simulink model "Const_VF_WithSlipCompensation"  (R2023a)
settings: Solver=VariableStepAuto  StartTime=0.0  StopTime=10.0  RelTol=1e-3
values from neighbouring files (symbols this model uses):
  Lm = .2037    (= 0.2037)    [Parameters.m]
  offset = Vph_p-(slope*Freq)    [Parameters.m]
  P = 4    [Parameters.m]
  slope = (Vph_p-VF_boost)/(Freq-1)    [Parameters.m]
  Te_rated = Prated/Wr_rated    (= 20.3536435794)    [Parameters.m]
  Vph_p = VLL_p/sqrt(3)    [Parameters.m]
  Wslip_rated = Ws_rated-Wr_rated    (= 5.23598775598)    [Parameters.m]
libraries: spsMosfetLib x6, spsabctodq0Lib x2, spsAsynchronousMachineSIUnitsLib x1, spsCurrentMeasurementLib x1, spsDCVoltageSourceLib x1, spsTriangleGeneratorLib x1, sps_lib x1
settings Model: Creator=User  LastModifiedBy=User

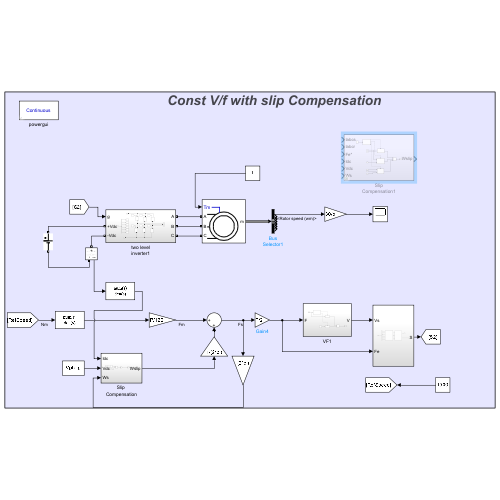
[thumbnail: Simulink's stored preview of the top-level diagram]
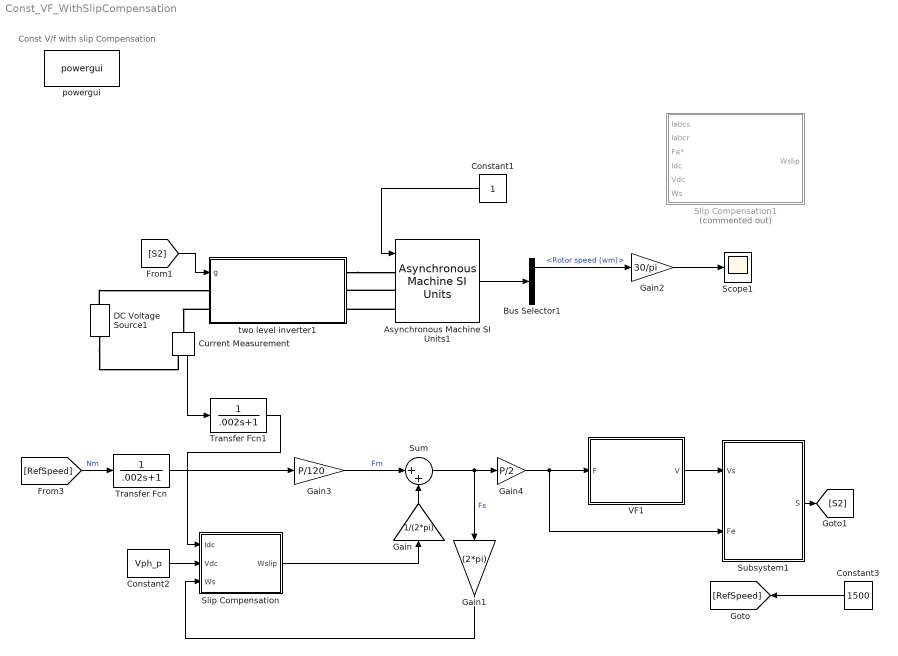
== system Const_VF_WithSlipCompensation ==
  note: Const V/f with slip Compensation
  Asynchronous Machine SI Units1 : spsAsynchronousMachineSIUnitsLib/Asynchronous Machine SI Units  RotorType=Squirrel-cage  PresetModel="01:  5 HP   460 V 60Hz 1750 RPM"  MechanicalLoad=Torque Tm  ShowDetailedParameters=on  ReferenceFrame=Stationary  Units=SI  MeasurementBus=off  NominalParameters=[3730 460 60]  VoltageRatio=1  Stator=[1.115 0.005974]  Rotor=[1.083 0.005974]  Cage1=[0.4155 0.002066]  Cage2=[0.4168 0.0003495]  Lm=0.2037  Mechanical=[0.02 0.005752 2]  PolePairs=2  InitialConditions=[1 0 0 0 0 0 0 0]  SimulateSaturation=off  Saturation=[14.03593122, 27.81365428, 53.79336849, 72.68890987, 97.98006896, 148.6815601, 215.7428561, 302.9841135, 428.7778367 ; 230, 322, 414, 460, 506, 552, 598, 644, 690]  LoadFlowParameters=1492000  TsPowergui=0  TsBlock=-1  IterativeModel=Trapezoidal non iterative  IterativeDiscreteModel=Trapezoidal non iterative  Pmec=1.492e+006
  Bus Selector1 : BusSelector  OutputSignals=Mechanical.Rotor speed (wm),Stator measurements.Stator current is_a (A),Stator measurements.Stator current is_b (A),Stator measurements.Stator current is_c (A),Rotor measurements.Rotor current ir_a (A),Rotor measurements.Rotor current ir_b (A),Rotor measurements.Rotor current ir_c (A)
  Constant1 : Constant
  Constant2 : Constant  Value=Vph_p
  Constant3 : Constant  Value=1500
  Current Measurement : spsCurrentMeasurementLib/Current Measurement  PhasorSimulation=off  OutputType=Complex  PSBequivalent=0
  DC Voltage Source1 : spsDCVoltageSourceLib/DC Voltage Source  Amplitude=Vph_p  Measurements=None
  Gain : Gain  Gain=1/(2*pi)
  Gain1 : Gain  Gain=(2*pi)
  Gain2 : Gain  Gain=30/pi
  Gain3 : Gain  Gain=P/120
  Gain4 : Gain  Gain=P/2
  Scope1 : Scope
  Slip Compensation1 : Subsystem  Commented=on
  Slip Compensation : Subsystem
  Subsystem1 : Subsystem
  Sum : Sum  Inputs=|++
  Transfer Fcn : TransferFcn  Denominator=[.002 1]
  Transfer Fcn1 : TransferFcn  Denominator=[.002 1]
  VF1 : Subsystem
  powergui : sps_lib/powergui  Priority=1  SimulationMode=Continuous  SampleTime=50e-6  frequency=60  Iterations=50  frequencyindice=60  Pbase=100e6  ErrMax=1e-4  UnitsV=kV  UnitsW=MW  buscounter=0  FunctionMessages=off  echomessages=off  EnableUseOfTLC=off  CurrentSourceSwitches=off  DisableSnubberDevices=off  DisableRonSwitches=off  DisableVfSwitches=off  DisplayEquations=off  AutomaticDiscreteSolvers=off  SolverType=Tustin/Backward Euler (TBE)  Interpol=off  ExternalGateDelay=off  methode=off  Ts=100  x0status=blocks  SPID=on  SwTol=0  HookPort=off  NonlinearTolerance=1e-4  nMaxIteration=100  ContinueOnMaxIteration=off  RestoreLinks=warning  ResistiveCurrentMeasurement=off  Frange=[0:2:500]  Ylog=off  Xlog=on  ShowGrid=off  save=off  variable=ZData  structure=0  ZoomFFT=off  StartTime=0.0  cycles=1  DisplayStyle=1  fundamental=60  FreqAxis=off  MaxFrequency=1000  frequencyindicesteady=1  RmsSteady=1  display=off
  two level inverter1 : Subsystem
  wires:
  Subsystem1/1(S) -> [S2]
  Gain3/1 -> Sum/1  "Fm"
  Gain2/1 -> Scope1/1
  Constant1/1 -> Asynchronous Machine SI Units1/1
  Sum/1 -> Gain4/1, Gain1/1  "Fs"
  [RefSpeed] -> Transfer Fcn/1  "Nm"
  [S2] -> two level inverter1/1(g)
  Asynchronous Machine SI Units1/1 -> Bus Selector1/1
  Bus Selector1/1 -> Gain2/1  "<Rotor speed (wm)>"
  VF1/1(V) -> Subsystem1/1(Vs)
  Constant3/1 -> [RefSpeed]
  Gain/1 -> Sum/2
  Gain4/1 -> Subsystem1/2(Fe), VF1/1(F)
  Transfer Fcn/1 -> Gain3/1
  Constant2/1 -> Slip Compensation/2(Vdc)
  Current Measurement/1 -> Transfer Fcn1/1
  Gain1/1 -> Slip Compensation/3(Ws)
  Transfer Fcn1/1 -> Slip Compensation/1(Idc)
  Slip Compensation/1(Wslip) -> Gain/1
  connections:
  DC Voltage Source1/RConn1 -- two level inverter1/LConn1
  two level inverter1/RConn1 -- Asynchronous Machine SI Units1/LConn1
  Asynchronous Machine SI Units1/LConn3 -- two level inverter1/RConn3
  DC Voltage Source1/LConn1 -- Current Measurement/RConn1
  Asynchronous Machine SI Units1/LConn2 -- two level inverter1/RConn2
  two level inverter1/LConn2 -- Current Measurement/LConn1

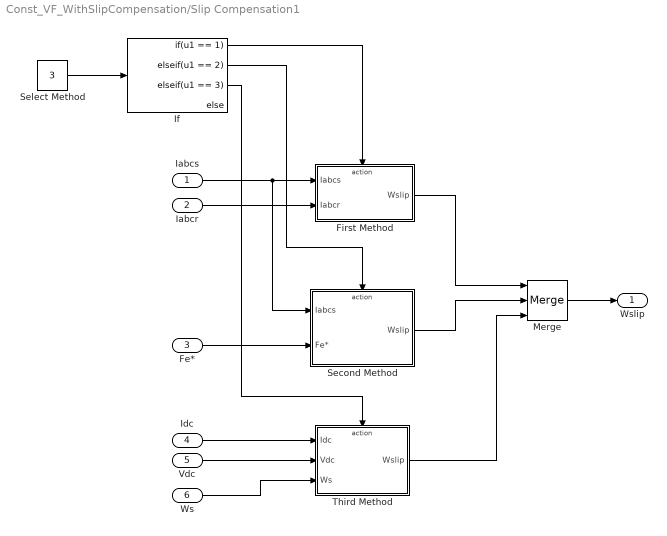
== system Const_VF_WithSlipCompensation/Slip Compensation1 ==
  Iabcs : Inport
  Iabcr : Inport  Port=2
  Fe* : Inport  Port=3
  Idc : Inport  Port=4
  Vdc : Inport  Port=5
  Ws : Inport  Port=6
  First Method : Subsystem  TreatAsAtomicUnit=on
  If : If  IfExpression=u1 == 1  ElseIfExpressions=u1 == 2,u1 == 3
  Merge : Merge  Inputs=3
  Second Method : Subsystem  TreatAsAtomicUnit=on
  Select Method : Constant  Value=3
  Third Method : Subsystem  TreatAsAtomicUnit=on
  Wslip : Outport
  wires:
  Ws/1 -> Third Method/3(Ws)
  Vdc/1 -> Third Method/2(Vdc)
  Idc/1 -> Third Method/1(Idc)
  Third Method/1(Wslip) -> Merge/3
  If/3 -> Third Method/Action
  Fe*/1 -> Second Method/2(Fe*)
  If/2 -> Second Method/Action
  Second Method/1(Wslip) -> Merge/2
  Merge/1 -> Wslip/1
  First Method/1(Wslip) -> Merge/1
  Iabcr/1 -> First Method/2(Iabcr)
  Iabcs/1 -> First Method/1(Iabcs), Second Method/1(Iabcs)
  If/1 -> First Method/Action
  Select Method/1 -> If/1

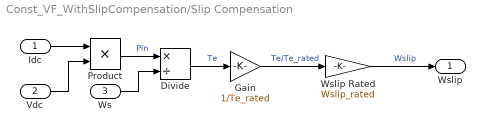
== system Const_VF_WithSlipCompensation/Slip Compensation ==
  Idc : Inport
  Vdc : Inport  Port=2
  Ws : Inport  Port=3
  Divide : Product  Inputs=*/
  Gain : Gain  Gain=1/Te_rated
  Product : Product
  Wslip Rated : Gain  Gain=Wslip_rated
  Wslip : Outport
  wires:
  Vdc/1 -> Product/2
  Product/1 -> Divide/1  "Pin"
  Ws/1 -> Divide/2
  Divide/1 -> Gain/1  "Te"
  Gain/1 -> Wslip Rated/1  "Te/Te_rated"
  Wslip Rated/1 -> Wslip/1  "Wslip"
  Idc/1 -> Product/1

== system Const_VF_WithSlipCompensation/Subsystem1 ==
  Vs : Inport
  Fe : Inport  Port=2
  Mux2 : Mux  Inputs=6
  SPWM2 : Subsystem
  Subsystem4 : Subsystem
  S : Outport
  wires:
  Subsystem4/3(Vc*) -> SPWM2/3(Vc*)
  SPWM2/3(S3) -> Mux2/3
  SPWM2/2(S2) -> Mux2/2
  SPWM2/1(S1) -> Mux2/1
  SPWM2/4(S4) -> Mux2/4
  SPWM2/6(S6) -> Mux2/6
  Subsystem4/1(Va*) -> SPWM2/1(Va*)
  Subsystem4/2(Vb*) -> SPWM2/2(Vb*)
  SPWM2/5(S5) -> Mux2/5
  Vs/1 -> Subsystem4/1(V_amp)
  Fe/1 -> Subsystem4/2(Frequency)
  Mux2/1 -> S/1

== system Const_VF_WithSlipCompensation/VF1 ==
  F : Inport
  Const Power : Subsystem  TreatAsAtomicUnit=on
  Const Torque : Subsystem  TreatAsAtomicUnit=on
  Constant : Constant  Value=Vph_p
  If : If  IfExpression=u1 <= 50
  Merge : Merge
  V : Outport
  wires:
  Const Power/1(Out1) -> Merge/2
  Constant/1 -> Const Power/1(In1)
  Merge/1 -> V/1
  If/1 -> Const Torque/Action
  Const Torque/1(Out1) -> Merge/1
  If/2 -> Const Power/Action
  F/1 -> If/1, Const Torque/1(F)

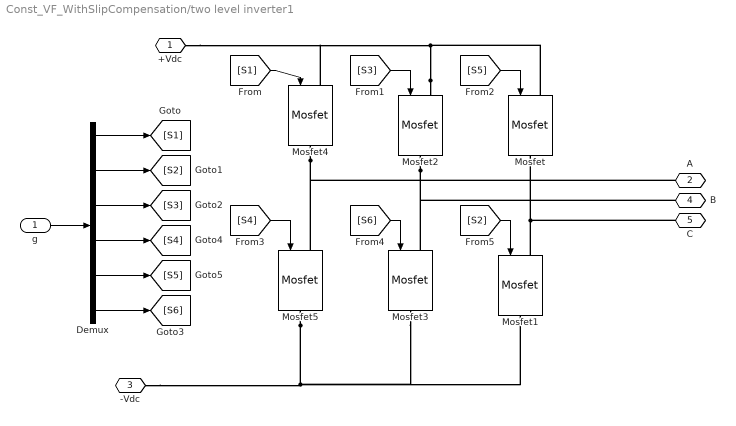
== system Const_VF_WithSlipCompensation/two level inverter1 ==
  g : Inport
  Demux : Demux  Outputs=6
  Mosfet{,1..5} (6 alike) : spsMosfetLib/Mosfet  Ron=0.1  Lon=0  Rd=0.01  Vfd=0  IC=0  Rs=1e5  Cs=inf  Measurements=off
  +Vdc : PMIOPort  Side=Left
  A : PMIOPort  Port=2  Side=Right
  -Vdc : PMIOPort  Port=3  Side=Left
  B : PMIOPort  Port=4  Side=Right
  C : PMIOPort  Port=5  Side=Right
  wires:
  [S2] -> Mosfet1/1
  [S6] -> Mosfet3/1
  [S4] -> Mosfet5/1
  [S5] -> Mosfet/1
  [S3] -> Mosfet2/1
  [S1] -> Mosfet4/1
  Demux/6 -> [S6]
  Demux/5 -> [S5]
  Demux/4 -> [S4]
  Demux/3 -> [S3]
  Demux/2 -> [S2]
  Demux/1 -> [S1]
  g/1 -> Demux/1
  connections:
  Mosfet4/RConn1 -- Mosfet5/LConn1 -- A/RConn1
  Mosfet2/RConn1 -- B/RConn1 -- Mosfet3/LConn1
  C/RConn1 -- Mosfet/RConn1 -- Mosfet1/LConn1
  Mosfet5/RConn1 -- -Vdc/RConn1 -- Mosfet1/RConn1 -- Mosfet3/RConn1
  Mosfet2/LConn1 -- Mosfet/LConn1 -- +Vdc/RConn1 -- Mosfet4/LConn1

== system Const_VF_WithSlipCompensation/Slip Compensation1/First Method ==
  Iabcs : Inport
  Iabcr : Inport  Port=2
  Action Port : ActionPort
  Subsystem : Subsystem
  Wslip : Outport
  wires:
  Iabcs/1 -> Subsystem/1(Iabcs)
  Iabcr/1 -> Subsystem/2(Iabcr)
  Subsystem/1(Wslip) -> Wslip/1

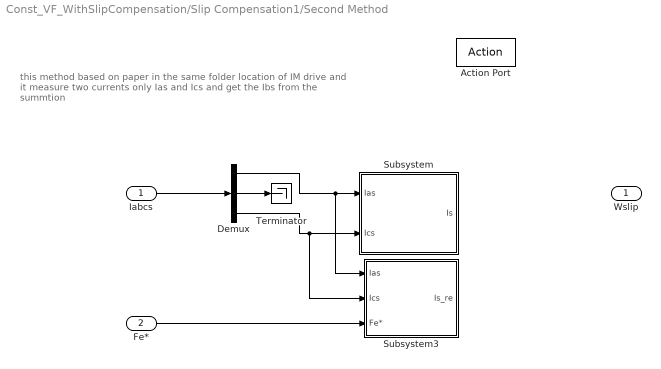
== system Const_VF_WithSlipCompensation/Slip Compensation1/Second Method ==
  note: this method based on paper in the same folder location of IM drive
      | and it measure two currents only Ias and Ics and get the Ibs from
      | the summtion
  Iabcs : Inport
  Fe* : Inport  Port=2
  Action Port : ActionPort
  Demux : Demux  Outputs=3
  Subsystem : Subsystem
  Subsystem3 : Subsystem
  Terminator : Terminator
  Wslip : Outport
  wires:
  Fe*/1 -> Subsystem3/3(Fe*)
  Demux/3 -> Subsystem/2(Ics), Subsystem3/2(Ics)
  Demux/2 -> Terminator/1
  Demux/1 -> Subsystem/1(Ias), Subsystem3/1(Ias)
  Iabcs/1 -> Demux/1

== system Const_VF_WithSlipCompensation/Slip Compensation1/Third Method ==
  Idc : Inport
  Vdc : Inport  Port=2
  Ws : Inport  Port=3
  Action Port : ActionPort
  Slip Compensation : Subsystem
  Wslip : Outport
  wires:
  Ws/1 -> Slip Compensation/3(Ws)
  Vdc/1 -> Slip Compensation/2(Vdc)
  Slip Compensation/1(Wslip) -> Wslip/1
  Idc/1 -> Slip Compensation/1(Idc)

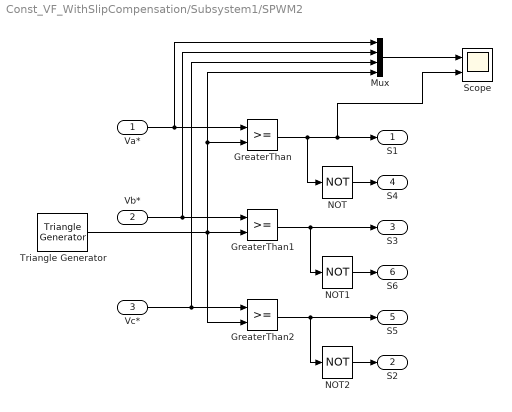
== system Const_VF_WithSlipCompensation/Subsystem1/SPWM2 ==
  Va* : Inport
  Vb* : Inport  Port=2
  Vc* : Inport  Port=3
  GreaterThan : RelationalOperator  OutDataTypeStr=boolean  RndMeth=Simplest  InputSameDT=off
  GreaterThan1 : RelationalOperator  OutDataTypeStr=boolean  RndMeth=Simplest  InputSameDT=off
  GreaterThan2 : RelationalOperator  OutDataTypeStr=boolean  RndMeth=Simplest  InputSameDT=off
  Mux : Mux
  NOT : Logic  Operator=NOT  IconShape=distinctive  AllPortsSameDT=off  OutDataTypeStr=boolean
  NOT1 : Logic  Operator=NOT  IconShape=distinctive  AllPortsSameDT=off  OutDataTypeStr=boolean
  NOT2 : Logic  Operator=NOT  IconShape=distinctive  AllPortsSameDT=off  OutDataTypeStr=boolean
  Scope : Scope  NumInputPorts=2
  Triangle Generator : spsTriangleGeneratorLib/Triangle Generator  Freq=5e3  Phase=90  Ts=0
  S1 : Outport
  S2 : Outport  Port=2
  S3 : Outport  Port=3
  S4 : Outport  Port=4
  S5 : Outport  Port=5
  S6 : Outport  Port=6
  wires:
  Mux/1 -> Scope/1
  NOT2/1 -> S2/1
  NOT1/1 -> S6/1
  NOT/1 -> S4/1
  GreaterThan2/1 -> S5/1, NOT2/1
  GreaterThan1/1 -> S3/1, NOT1/1
  GreaterThan/1 -> S1/1, Scope/2, NOT/1
  Vc*/1 -> GreaterThan2/1, Mux/3
  Vb*/1 -> GreaterThan1/1, Mux/2
  Va*/1 -> GreaterThan/1, Mux/1
  Triangle Generator/1 -> GreaterThan/2, Mux/4, GreaterThan1/2, GreaterThan2/2

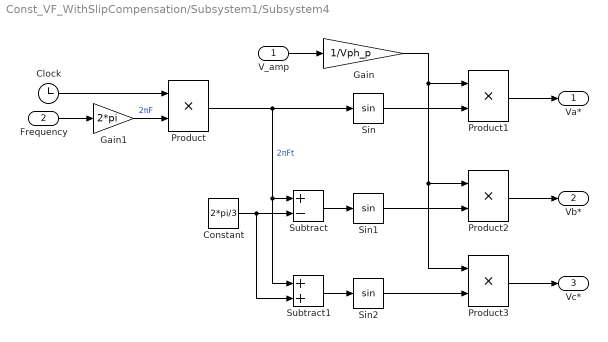
== system Const_VF_WithSlipCompensation/Subsystem1/Subsystem4 ==
  V_amp : Inport
  Frequency : Inport  Port=2
  Clock : Clock
  Constant : Constant  Value=2*pi/3
  Gain : Gain  Gain=1/Vph_p
  Gain1 : Gain  Gain=2*pi
  Product{,1..3} (4 alike) : Product
  Sin : Trigonometry
  Sin1 : Trigonometry
  Sin2 : Trigonometry
  Subtract : Sum  Inputs=+-
  Subtract1 : Sum
  Va* : Outport
  Vb* : Outport  Port=2
  Vc* : Outport  Port=3
  wires:
  Product3/1 -> Vc*/1
  Product2/1 -> Vb*/1
  Sin2/1 -> Product3/2
  Sin1/1 -> Product2/2
  Product1/1 -> Va*/1
  Gain/1 -> Product1/1, Product2/1, Product3/1
  Sin/1 -> Product1/2
  Constant/1 -> Subtract/2, Subtract1/2
  Subtract1/1 -> Sin2/1
  Subtract/1 -> Sin1/1
  Product/1 -> Sin/1, Subtract/1, Subtract1/1  "2πFt"
  Clock/1 -> Product/1
  Gain1/1 -> Product/2  "2πF"
  Frequency/1 -> Gain1/1
  V_amp/1 -> Gain/1

== system Const_VF_WithSlipCompensation/VF1/Const Power ==
  In1 : Inport
  Action Port : ActionPort  ActionPortLabel=else
  Out1 : Outport
  wires:
  In1/1 -> Out1/1

== system Const_VF_WithSlipCompensation/VF1/Const Torque ==
  F : Inport
  Action Port : ActionPort  ActionPortLabel=if(u1 <= 50)
  Add : Sum
  Constant : Constant  Value=offset
  Gain : Gain  Gain=slope
  Out1 : Outport
  wires:
  Constant/1 -> Add/2
  Add/1 -> Out1/1
  Gain/1 -> Add/1
  F/1 -> Gain/1

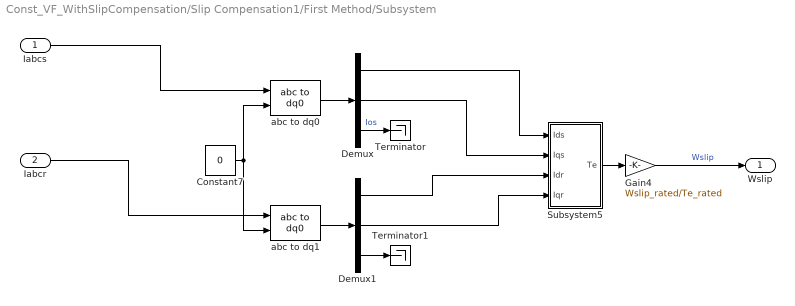
== system Const_VF_WithSlipCompensation/Slip Compensation1/First Method/Subsystem ==
  Iabcs : Inport
  Iabcr : Inport  Port=2
  Constant7 : Constant  Value=0
  Demux : Demux  Outputs=3
  Demux1 : Demux  Outputs=3
  Gain4 : Gain  Gain=Wslip_rated/Te_rated
  Subsystem5 : Subsystem
  Terminator : Terminator
  Terminator1 : Terminator
  abc to dq0 : spsabctodq0Lib/abc to dq0  Alignment=90 degrees behind phase A axis
  abc to dq1 : spsabctodq0Lib/abc to dq0  Alignment=90 degrees behind phase A axis
  Wslip : Outport
  wires:
  Gain4/1 -> Wslip/1  "Wslip"
  Iabcs/1 -> abc to dq0/1
  Iabcr/1 -> abc to dq1/1
  Demux1/3 -> Terminator1/1
  Demux/2 -> Subsystem5/2(Iqs)
  Demux1/1 -> Subsystem5/3(Idr)
  abc to dq1/1 -> Demux1/1
  Demux/3 -> Terminator/1  "Ios"
  abc to dq0/1 -> Demux/1
  Demux1/2 -> Subsystem5/4(Iqr)
  Demux/1 -> Subsystem5/1(Ids)
  Constant7/1 -> abc to dq0/2, abc to dq1/2
  Subsystem5/1(Te) -> Gain4/1

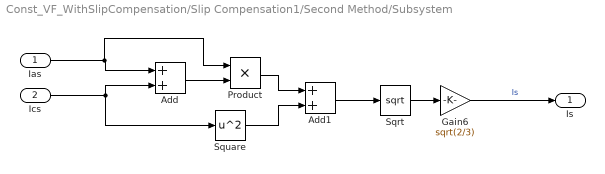
== system Const_VF_WithSlipCompensation/Slip Compensation1/Second Method/Subsystem ==
  Ias : Inport
  Ics : Inport  Port=2
  Add : Sum
  Add1 : Sum
  Gain6 : Gain  Gain=sqrt(2/3)
  Product : Product
  Sqrt : Sqrt
  Square : Math  Operator=square
  Is : Outport
  wires:
  Gain6/1 -> Is/1  "Is"
  Product/1 -> Add1/1
  Add1/1 -> Sqrt/1
  Ics/1 -> Square/1, Add/2
  Square/1 -> Add1/2
  Sqrt/1 -> Gain6/1
  Add/1 -> Product/2
  Ias/1 -> Add/1, Product/1

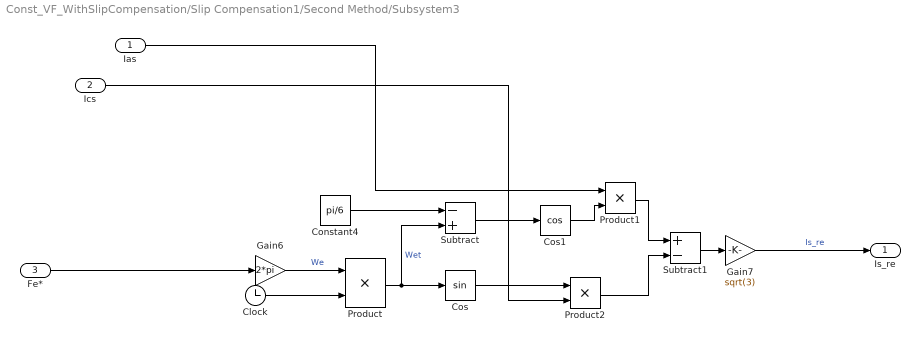
== system Const_VF_WithSlipCompensation/Slip Compensation1/Second Method/Subsystem3 ==
  Ias : Inport
  Ics : Inport  Port=2
  Fe* : Inport  Port=3
  Clock : Clock
  Constant4 : Constant  Value=pi/6
  Cos : Trigonometry
  Cos1 : Trigonometry  Operator=cos
  Gain6 : Gain  Gain=2*pi
  Gain7 : Gain  Gain=sqrt(3)
  Product : Product
  Product1 : Product
  Product2 : Product
  Subtract : Sum  Inputs=-+
  Subtract1 : Sum  Inputs=+-
  Is_re : Outport
  wires:
  Fe*/1 -> Gain6/1
  Gain7/1 -> Is_re/1  "Is_re"
  Ics/1 -> Product2/2
  Ias/1 -> Product1/1
  Subtract1/1 -> Gain7/1
  Cos/1 -> Product2/1
  Gain6/1 -> Product/1  "We"
  Subtract/1 -> Cos1/1
  Product1/1 -> Subtract1/1
  Product/1 -> Cos/1, Subtract/2  "Wet"
  Clock/1 -> Product/2
  Product2/1 -> Subtract1/2
  Cos1/1 -> Product1/2
  Constant4/1 -> Subtract/1

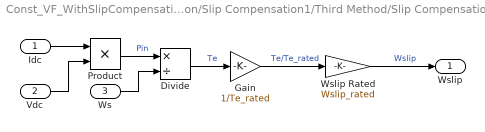
== system Const_VF_WithSlipCompensation/Slip Compensation1/Third Method/Slip Compensation ==
  Idc : Inport
  Vdc : Inport  Port=2
  Ws : Inport  Port=3
  Divide : Product  Inputs=*/
  Gain : Gain  Gain=1/Te_rated
  Product : Product
  Wslip Rated : Gain  Gain=Wslip_rated
  Wslip : Outport
  wires:
  Idc/1 -> Product/1
  Wslip Rated/1 -> Wslip/1  "Wslip"
  Gain/1 -> Wslip Rated/1  "Te/Te_rated"
  Divide/1 -> Gain/1  "Te"
  Ws/1 -> Divide/2
  Product/1 -> Divide/1  "Pin"
  Vdc/1 -> Product/2

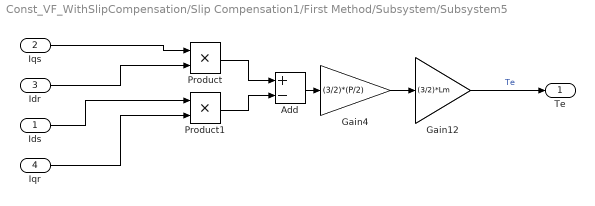
== system Const_VF_WithSlipCompensation/Slip Compensation1/First Method/Subsystem/Subsystem5 ==
  Ids : Inport
  Iqs : Inport  Port=2
  Idr : Inport  Port=3
  Iqr : Inport  Port=4
  Add : Sum  Inputs=+-
  Gain12 : Gain  Gain=(3/2)*Lm
  Gain4 : Gain  Gain=(3/2)*(P/2)
  Product : Product
  Product1 : Product
  Te : Outport
  wires:
  Iqs/1 -> Product/1
  Add/1 -> Gain4/1
  Idr/1 -> Product/2
  Gain12/1 -> Te/1  "Te"
  Product/1 -> Add/1
  Ids/1 -> Product1/1
  Product1/1 -> Add/2
  Gain4/1 -> Gain12/1
  Iqr/1 -> Product1/2
